simulink model "Averaged_nobattery"  (R2020a)
settings: Solver=VariableStepAuto  StartTime=0.0  StopTime=30  MaxStep=1e-2  RelTol=1e-3
undefined symbols (not defined in the file): CQ, I, Ke, Om, R, Ra, speedCmd, V0
libraries: fmu_me_lib x4, simulink x4
settings Model: Creator=Bob  LastModifiedBy=meagh
settings SFSimCC: CustomCodeUndefinedFunction=UseInterfaceOnly

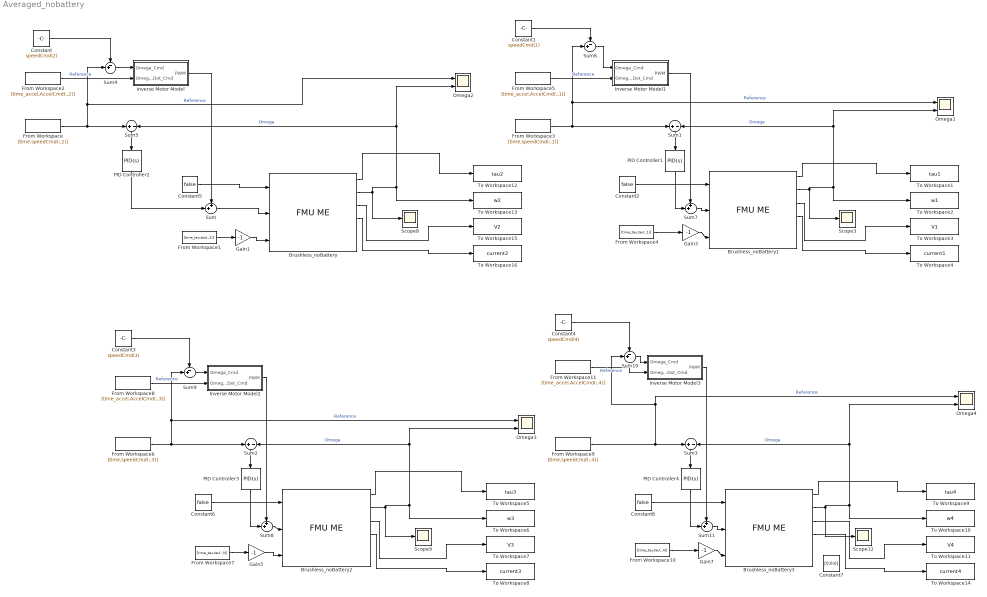
== system Averaged_nobattery ==
  Brushless_noBattery{,1..3} (4 alike) : fmu_me_lib/FMU ME  Description=Simulates an FMU for Model Exchange 1.0 or Model Exchange 2.0.  dummy=0
  Constant : Constant  Value=speedCmd(2)
  Constant1 : Constant  Value=speedCmd(1)
  Constant{2,5..6,8} (4 alike) : Constant  Value=false  OutDataTypeStr=boolean
  Constant3 : Constant  Value=speedCmd(3)
  Constant4 : Constant  Value=speedCmd(4)
  Constant7 : Constant  Value=[0;0;0]
  From Workspace : FromWorkspace  VariableName=[time,speedCmd(:,2)]
  From Workspace1 : FromWorkspace  VariableName=[time_tau,tau(:,2)]
  From Workspace10 : FromWorkspace  VariableName=[time_tau,tau(:,4)]
  From Workspace11 : FromWorkspace  VariableName=[time_accel,AccelCmd(:,4)]
  From Workspace2 : FromWorkspace  VariableName=[time_accel,AccelCmd(:,2)]
  From Workspace3 : FromWorkspace  VariableName=[time,speedCmd(:,1)]
  From Workspace4 : FromWorkspace  VariableName=[time_tau,tau(:,1)]
  From Workspace5 : FromWorkspace  VariableName=[time_accel,AccelCmd(:,1)]
  From Workspace6 : FromWorkspace  VariableName=[time,speedCmd(:,3)]
  From Workspace7 : FromWorkspace  VariableName=[time_tau,tau(:,3)]
  From Workspace8 : FromWorkspace  VariableName=[time_accel,AccelCmd(:,3)]
  From Workspace9 : FromWorkspace  VariableName=[time,speedCmd(:,4)]
  Gain{1,3,5,7} (4 alike) : Gain  Gain=-1
  Inverse Motor Model : Subsystem
  Inverse Motor Model1 : Subsystem
  Inverse Motor Model2 : Subsystem
  Inverse Motor Model3 : Subsystem
  Omega{1..4} (4 alike) : Scope  NumInputPorts=2
  PID Controller{1..4} (4 alike) : simulink/Continuous/PID Controller  Controller=PID  Form=Parallel  TimeDomain=Continuous-time  UseExternalTs=off  SampleTime=-1  IntegratorMethod=Forward Euler  FilterMethod=Forward Euler  ControllerParametersSource=internal  P=0.0184*0.2  I=0.0184  D=0  UseFilter=on  N=100  TunerSelectOption=Transfer Function Based (PID Tuner App)  InitialConditionSource=internal  InitialConditionForIntegrator=0  InitialConditionForFilter=0  DifferentiatorICPrevScaledInput=0  ExternalReset=none  TrackingMode=off  Kt=1  LimitOutput=off  UpperSaturationLimit=inf  LowerSaturationLimit=-inf  LinearizeAsGain=on  AntiWindupMode=none  Kb=1  POutMin=[]  POutMax=[]  IOutMin=[]  IOutMax=[]  DOutMin=[]  DOutMax=[]  NOutMin=[]  NOutMax=[]  SumOutMin=[]  SumOutMax=[]  SaturationOutMin=[]  SaturationOutMax=[]  PParamMin=[]  PParamMax=[]  IParamMin=[]  IParamMax=[]  DParamMin=[]  DParamMax=[]  NParamMin=[]  NParamMax=[]  KbParamMin=[]  KbParamMax=[]  KtParamMin=[]  KtParamMax=[]  KbOutMin=[]  KbOutMax=[]  KtOutMin=[]  KtOutMax=[]  IntegratorOutMin=[]  IntegratorOutMax=[]  FilterOutMin=[]  FilterOutMax=[]  SumI1OutMin=[]  SumI1OutMax=[]  SumI2OutMin=[]  SumI2OutMax=[]  SumI3OutMin=[]  SumI3OutMax=[]  SumI4OutMin=[]  SumI4OutMax=[]  SumDOutMin=[]  SumDOutMax=[]  DifferentiatorOutMin=[]  DifferentiatorOutMax=[]  FilterDiffOutCoefMin=[]  FilterDiffOutCoefMax=[]  ReciprocalOutMin=[]  ReciprocalOutMax=[]  SumDenOutMin=[]  SumDenOutMax=[]  SumNumOutMin=[]  SumNumOutMax=[]  DivideOutMin=[]  DivideOutMax=[]  UdiffTsProdOutMin=[]  UdiffTsProdOutMax=[]  NTsProdOutMin=[]  NTsProdOutMax=[]  UintegralTsProdOutMin=[]  UintegralTsProdOutMax=[]  UngainTsProdOutMin=[]  UngainTsProdOutMax=[]  IntegratorContinuousStateAttributes=''  IntegratorStateMustResolveToSignalObject=off  IntegratorRTWStateStorageClass=Auto  FilterContinuousStateAttributes=''  FilterStateMustResolveToSignalObject=off  FilterRTWStateStorageClass=Auto  ParallelPVariant=InternalParameters  IdealPVariant=Disabled  IVariant=InternalParameters  DVariant=InternalParameters  IntegratorVariant=Continuous  SatVariant=Disabled  AWVariant=Passthrough  PCopyVariant=Disabled  TRVariant=Disabled  FdbkBlocksVariant=Forward  IdealPFdbkVariant=Disabled  SatFdbkVariant=Disabled  DerivativeFilterVariant=ContFilter  NVariant=InternalParameters  NCopyVariant=Disabled  FilterICVariant=InternalICsFilter  IntegratorICVariant=InternalICs  ExternalResetVariant=Disabled  TRSumVariant=Passthrough  SumFdbkVariant=Disabled  SumVariant=Sum_PID  TsampFilterVariant=InternalTs  TsampNgainVariant=Passthrough  TsampIntegralVariant=Passthrough
  Scope{3,8..9,12} (4 alike) : Scope
  Sum{,7..8,11} (4 alike) : Sum  Inputs=++|
  Sum{1..3,5} (4 alike) : Sum  Inputs=+|-
  Sum{4,6,9..10} (4 alike) : Sum  Inputs=-+|
  To Workspace1 : ToWorkspace  VariableName=tau1  SaveFormat=Timeseries  SampleTime=-1
  To Workspace10 : ToWorkspace  VariableName=w4  SaveFormat=Timeseries  SampleTime=-1
  To Workspace11 : ToWorkspace  VariableName=V4  SaveFormat=Timeseries  SampleTime=-1
  To Workspace12 : ToWorkspace  VariableName=tau2  SaveFormat=Timeseries  SampleTime=-1
  To Workspace13 : ToWorkspace  VariableName=w2  SaveFormat=Timeseries  SampleTime=-1
  To Workspace14 : ToWorkspace  VariableName=current4  SaveFormat=Timeseries  SampleTime=-1
  To Workspace15 : ToWorkspace  VariableName=V2  SaveFormat=Timeseries  SampleTime=-1
  To Workspace16 : ToWorkspace  VariableName=current2  SaveFormat=Timeseries  SampleTime=-1
  To Workspace2 : ToWorkspace  VariableName=w1  SaveFormat=Timeseries  SampleTime=-1
  To Workspace3 : ToWorkspace  VariableName=V1  SaveFormat=Timeseries  SampleTime=-1
  To Workspace4 : ToWorkspace  VariableName=current1  SaveFormat=Timeseries  SampleTime=-1
  To Workspace5 : ToWorkspace  VariableName=tau3  SaveFormat=Timeseries  SampleTime=-1
  To Workspace6 : ToWorkspace  VariableName=w3  SaveFormat=Timeseries  SampleTime=-1
  To Workspace7 : ToWorkspace  VariableName=V3  SaveFormat=Timeseries  SampleTime=-1
  To Workspace8 : ToWorkspace  VariableName=current3  SaveFormat=Timeseries  SampleTime=-1
  To Workspace9 : ToWorkspace  VariableName=tau4  SaveFormat=Timeseries  SampleTime=-1
  wires:
  Constant5/1 -> Brushless_noBattery/1
  Brushless_noBattery/1 -> To Workspace12/1
  Brushless_noBattery/4 -> To Workspace16/1
  Brushless_noBattery/3 -> To Workspace15/1
  Brushless_noBattery/2 -> To Workspace13/1, Sum5/2, Omega2/2, Scope8/1  "Omega"
  Sum5/1 -> PID Controller2/1
  From Workspace1/1 -> Gain1/1
  Gain1/1 -> Brushless_noBattery/3
  Gain3/1 -> Brushless_noBattery1/3
  Brushless_noBattery1/2 -> To Workspace2/1, Omega1/2, Sum1/2, Scope3/1  "Omega"
  Brushless_noBattery1/3 -> To Workspace3/1
  Brushless_noBattery1/1 -> To Workspace1/1
  Sum1/1 -> PID Controller1/1
  Constant2/1 -> Brushless_noBattery1/1
  Brushless_noBattery1/4 -> To Workspace4/1
  From Workspace4/1 -> Gain3/1
  Brushless_noBattery2/2 -> To Workspace6/1, Omega3/2, Sum2/2, Scope9/1  "Omega"
  Gain5/1 -> Brushless_noBattery2/3
  From Workspace7/1 -> Gain5/1
  Brushless_noBattery2/4 -> To Workspace8/1
  Sum2/1 -> PID Controller3/1
  Brushless_noBattery2/3 -> To Workspace7/1
  Brushless_noBattery2/1 -> To Workspace5/1
  Constant6/1 -> Brushless_noBattery2/1
  Brushless_noBattery3/2 -> To Workspace10/1, Omega4/2, Sum3/2, Scope12/1  "Omega"
  Gain7/1 -> Brushless_noBattery3/3
  From Workspace10/1 -> Gain7/1
  Brushless_noBattery3/4 -> To Workspace14/1
  Sum3/1 -> PID Controller4/1
  Brushless_noBattery3/3 -> To Workspace11/1
  Brushless_noBattery3/1 -> To Workspace9/1
  Constant8/1 -> Brushless_noBattery3/1
  From Workspace/1 -> Omega2/1, Sum4/2, Sum5/1  "Reference"
  From Workspace2/1 -> Inverse Motor Model/2(OmegaDot_Cmd)  "Reference"
  PID Controller2/1 -> Sum/2
  Sum/1 -> Brushless_noBattery/2
  Inverse Motor Model/1(PWM) -> Sum/1
  Sum4/1 -> Inverse Motor Model/1(Omega_Cmd)
  Constant/1 -> Sum4/1
  From Workspace5/1 -> Inverse Motor Model1/2(OmegaDot_Cmd)  "Reference"
  Constant1/1 -> Sum6/1
  From Workspace3/1 -> Sum1/1, Sum6/2, Omega1/1  "Reference"
  Sum6/1 -> Inverse Motor Model1/1(Omega_Cmd)
  Inverse Motor Model1/1(PWM) -> Sum7/1
  PID Controller1/1 -> Sum7/2
  Sum7/1 -> Brushless_noBattery1/2
  PID Controller3/1 -> Sum8/2
  Sum8/1 -> Brushless_noBattery2/2
  From Workspace6/1 -> Sum2/1, Sum9/2, Omega3/1  "Reference"
  Sum9/1 -> Inverse Motor Model2/1(Omega_Cmd)
  Constant3/1 -> Sum9/1
  From Workspace8/1 -> Inverse Motor Model2/2(OmegaDot_Cmd)  "Reference"
  Inverse Motor Model2/1(PWM) -> Sum8/1
  Sum10/1 -> Inverse Motor Model3/1(Omega_Cmd)
  From Workspace11/1 -> Inverse Motor Model3/2(OmegaDot_Cmd)  "Reference"
  From Workspace9/1 -> Omega4/1, Sum10/2, Sum3/1  "Reference"
  Constant4/1 -> Sum10/1
  Inverse Motor Model3/1(PWM) -> Sum11/1
  Sum11/1 -> Brushless_noBattery3/2
  PID Controller4/1 -> Sum11/2

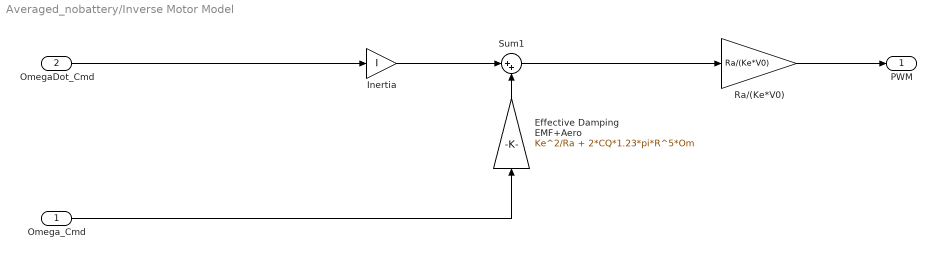
== system Averaged_nobattery/Inverse Motor Model ==
  Omega_Cmd : Inport
  OmegaDot_Cmd : Inport  Port=2
  Effective Damping EMF+Aero : Gain  Gain=Ke^2/Ra + 2*CQ*1.23*pi*R^5*Om
  Inertia : Gain  Gain=I
  Ra/(Ke*V0) : Gain  Gain=Ra/(Ke*V0)
  Sum1 : Sum  Inputs=|++
  PWM : Outport  VectorParamsAs1DForOutWhenUnconnected=off
  wires:
  Ra/(Ke*V0)/1 -> PWM/1
  Sum1/1 -> Ra/(Ke*V0)/1
  Effective Damping EMF+Aero/1 -> Sum1/2
  Inertia/1 -> Sum1/1
  Omega_Cmd/1 -> Effective Damping EMF+Aero/1
  OmegaDot_Cmd/1 -> Inertia/1

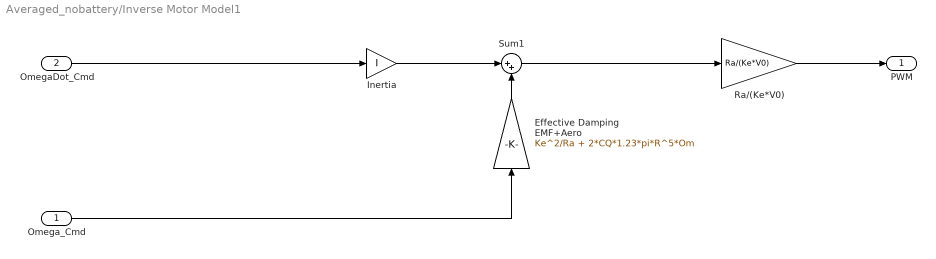
== system Averaged_nobattery/Inverse Motor Model1 ==
  Omega_Cmd : Inport
  OmegaDot_Cmd : Inport  Port=2
  Effective Damping EMF+Aero : Gain  Gain=Ke^2/Ra + 2*CQ*1.23*pi*R^5*Om
  Inertia : Gain  Gain=I
  Ra/(Ke*V0) : Gain  Gain=Ra/(Ke*V0)
  Sum1 : Sum  Inputs=|++
  PWM : Outport  VectorParamsAs1DForOutWhenUnconnected=off
  wires:
  Ra/(Ke*V0)/1 -> PWM/1
  Sum1/1 -> Ra/(Ke*V0)/1
  Effective Damping EMF+Aero/1 -> Sum1/2
  Inertia/1 -> Sum1/1
  Omega_Cmd/1 -> Effective Damping EMF+Aero/1
  OmegaDot_Cmd/1 -> Inertia/1

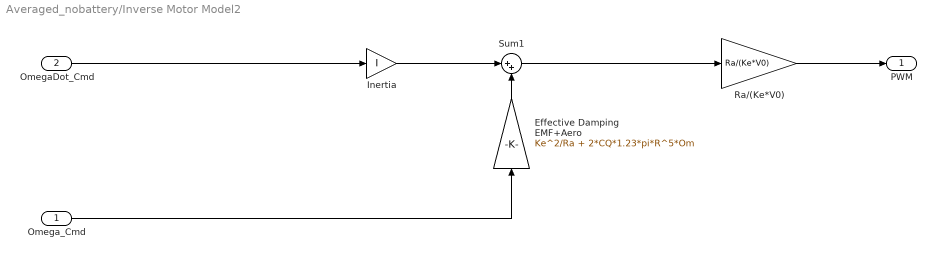
== system Averaged_nobattery/Inverse Motor Model2 ==
  Omega_Cmd : Inport
  OmegaDot_Cmd : Inport  Port=2
  Effective Damping EMF+Aero : Gain  Gain=Ke^2/Ra + 2*CQ*1.23*pi*R^5*Om
  Inertia : Gain  Gain=I
  Ra/(Ke*V0) : Gain  Gain=Ra/(Ke*V0)
  Sum1 : Sum  Inputs=|++
  PWM : Outport  VectorParamsAs1DForOutWhenUnconnected=off
  wires:
  Ra/(Ke*V0)/1 -> PWM/1
  Sum1/1 -> Ra/(Ke*V0)/1
  Effective Damping EMF+Aero/1 -> Sum1/2
  Inertia/1 -> Sum1/1
  Omega_Cmd/1 -> Effective Damping EMF+Aero/1
  OmegaDot_Cmd/1 -> Inertia/1

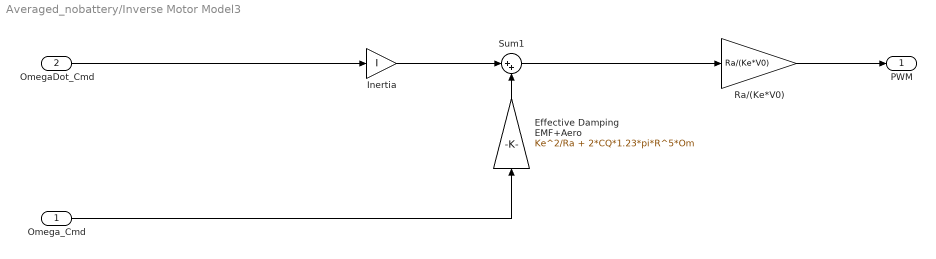
== system Averaged_nobattery/Inverse Motor Model3 ==
  Omega_Cmd : Inport
  OmegaDot_Cmd : Inport  Port=2
  Effective Damping EMF+Aero : Gain  Gain=Ke^2/Ra + 2*CQ*1.23*pi*R^5*Om
  Inertia : Gain  Gain=I
  Ra/(Ke*V0) : Gain  Gain=Ra/(Ke*V0)
  Sum1 : Sum  Inputs=|++
  PWM : Outport  VectorParamsAs1DForOutWhenUnconnected=off
  wires:
  Ra/(Ke*V0)/1 -> PWM/1
  Sum1/1 -> Ra/(Ke*V0)/1
  Effective Damping EMF+Aero/1 -> Sum1/2
  Inertia/1 -> Sum1/1
  Omega_Cmd/1 -> Effective Damping EMF+Aero/1
  OmegaDot_Cmd/1 -> Inertia/1
